simulink model "sim_syst"  (R2025b)
settings: Solver=VariableStepAuto  StartTime=0.0  StopTime=10.0  RelTol=1e-3
settings Model: Creator=Armando  LastModifiedBy=Armando

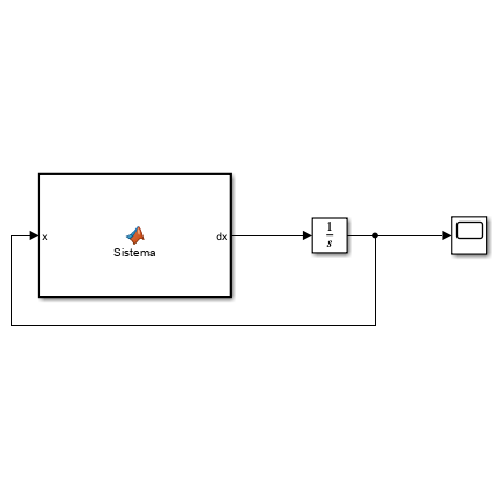
[thumbnail: Simulink's stored preview of the top-level diagram]
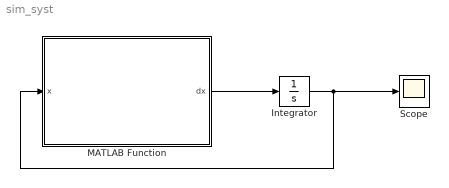
== system sim_syst ==
  Integrator : Integrator  InitialCondition=1
  MATLAB Function : MATLAB Function  TreatAsAtomicUnit=on
  Scope : Scope
      settings: ActiveDisplayYMinimum=-16.992531687443218  ActiveDisplayYMaximum=137.01845912002364
  wires:
  MATLAB Function/1(dx) -> Integrator/1
  Integrator/1 -> MATLAB Function/1(x), Scope/1

== matlab function sim_syst/MATLAB Function ==
  data: x input; dx output
function dx = Sistema(x)
dx = x^3;
